simulink model "LR6"  (R2021a)
settings: Solver=VariableStepAuto  StartTime=0.0  StopTime=10.0  RelTol=1e-3
settings Model: Creator=Rubina  LastModifiedBy=Rubina

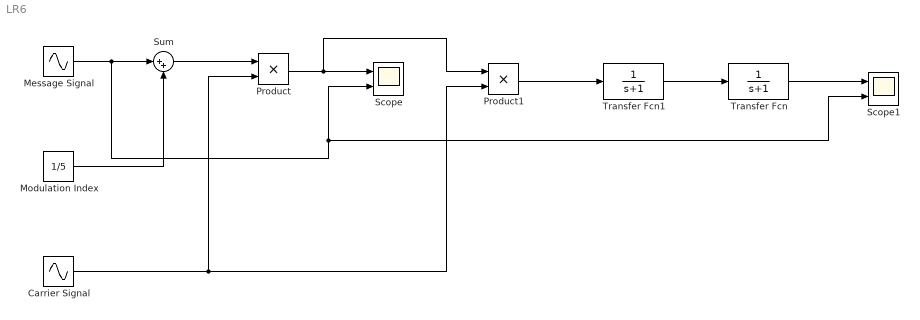
== system LR6 ==
  Carrier Signal : Sin  Amplitude=5  Frequency=2*pi*10  SampleTime=1/8000
  Message Signal : Sin  Frequency=2*pi  SampleTime=1/8000
  Modulation Index : Constant  Value=1/5  SampleTime=1/8000
  Product : Product
  Product1 : Product
  Scope : Scope  NumInputPorts=2
  Scope1 : Scope  NumInputPorts=2
  Sum : Sum  Inputs=|++
  Transfer Fcn : TransferFcn  Denominator=[1 1]
  Transfer Fcn1 : TransferFcn  Denominator=[1 1]
  wires:
  Sum/1 -> Product/1
  Product/1 -> Product1/1, Scope/1
  Product1/1 -> Transfer Fcn1/1
  Transfer Fcn1/1 -> Transfer Fcn/1
  Transfer Fcn/1 -> Scope1/1
  Message Signal/1 -> Scope1/2, Scope/2, Sum/1
  Carrier Signal/1 -> Product/2, Product1/2
  Modulation Index/1 -> Sum/2
